simulink model "modelo_f_EXPORT_TO_CODESYS"  (R2024b)
settings: Solver=FixedStepAuto  StartTime=0.0  StopTime=inf  FixedStep=0.001  RelTol=1e-3  EnableMultiTasking=on
InitFcn:
  | clc
  | clear
  | close all
  | clear all
  | clear mex
  | parametros
  | gain_CL
  | calculo_observador_carro
  | calculo_observador_izaje
values from neighbouring files (symbols this model uses):
  b_cx = 1e6    (= 1000000)    [parametros.m]
  b_cy = 1e7    (= 10000000)    [parametros.m]
  b_hb = 1e8    (= 100000000)    [parametros.m]
  b_hd = 8    [parametros.m]
  b_hm = 18    [parametros.m]
  b_t = 90    [parametros.m]
  b_tb = 5e6    (= 5000000)    [parametros.m]
  b_td = 1.8    [parametros.m]
  b_tm = 6    [parametros.m]
  b_tw = 3e3    (= 3000)    [parametros.m]
  b_wu = 150    [parametros.m]
  container_pillars = container_pillars(randperm(19))    [parametros.m]
  dx_grid_lidar = 0.01    [parametros.m]
  escenario = 1    [parametros.m]
  g = 9.80665    [parametros.m]
  H_c = 2.59    [parametros.m]
  H_truck = 1    [parametros.m]
  i_h = 22    [parametros.m]
  i_t = 30    [parametros.m]
  J_hd_hEb = 3800    [parametros.m]
  J_hm_hb = 30    [parametros.m]
  J_td = 1200    [parametros.m]
  J_tm_tb = 7    [parametros.m]
  K_cy = 1.8e9    (= 1800000000)    [parametros.m]
  K_tw = 4.8e5    (= 480000)    [parametros.m]
  k_wu = 2.36e8    (= 236000000)    [parametros.m]
  l_h0 = (Y_t0-y_l0)    (= 38)    [parametros.m]
  l_h_max = Y_t0-y_h_min    (= 65)    [parametros.m]
  l_h_maxE = l_h_max+0.5    (= 65.5)    [parametros.m]
  l_h_min = Y_t0-y_h_max    (= 5)    [parametros.m]
  l_h_minE = l_h_min-0.5    (= 4.5)    [parametros.m]
  M_cmax = 50000    [parametros.m]
  M_cmin = 2000    [parametros.m]
  M_s = 15000    [parametros.m]
  M_t = 30000    [parametros.m]
  r_hd = 0.75    [parametros.m]
  r_td = 0.50    (= 0.5)    [parametros.m]
  T_hbMax = 5e4    (= 50000)    [parametros.m]
  T_hEbMax = 1.1e6    (= 1100000)    [parametros.m]
  T_hmMax = 2e4    (= 20000)    [parametros.m]
  T_s = 0.001    [parametros.m]
  T_s0 = 0.001    [parametros.m]
  T_s1 = 0.020    (= 0.02)    [parametros.m]
  T_s2 = 0.020    (= 0.02)    [parametros.m]
  T_tbMax = 5e3    (= 5000)    [parametros.m]
  T_tmMax = 4e3    (= 4000)    [parametros.m]
  tau_tm = 1e-3    (= 0.001)    [parametros.m]
  theta_hm0 = -l_h0*i_h*2/r_hd    (= -2229.33333333)    [parametros.m]
  theta_tm0 = (x_t0)*i_t/r_td    (= -900)    [parametros.m]
  trucks0 = [0, 0, 0, 0, 0]    [parametros.m]
  v_h_max_load = 1.5    [parametros.m]
  v_h_max_noload = 3    [parametros.m]
  v_lx0 = 0    [parametros.m]
  v_ly0 = 0    [parametros.m]
  v_t0 = 0    [parametros.m]
  v_t_max = 4    [parametros.m]
  W_c = ctrb(A, B_c(:,1))    [CyO_carro.m]    (also in CyO_izaje.m; parametros.m = 2.44)
  w_hm0 = 0    [parametros.m]
  w_hm_min_BRK = 0.005    [parametros.m]
  w_hm_rated = v_h_max_load*2*i_h/r_hd    (= 88)    [parametros.m]
  w_tm0 = (v_t0)*i_t/r_td    (= 0)    [parametros.m]
  w_tm_min_BRK = 0.005    [parametros.m]
  x_c0_left = -35    [parametros.m]
  x_c0_right = 55    [parametros.m]
  x_containers_left_lim = 1.5    [parametros.m]
  x_containers_right_lim = 48.5    [parametros.m]
  x_l0 = x_t0    (= -15)    [parametros.m]
  x_lidar_offset = 3.0    (= 3)    [parametros.m]
  x_t0 = -15    [parametros.m]
  x_t_max = 50    [parametros.m]
  x_t_maxE = x_t_max+0.5    (= 50.5)    [parametros.m]
  x_t_min = -30    [parametros.m]
  x_t_minE = x_t_min-0.5    (= -30.5)    [parametros.m]
  y_h_min = -20    [parametros.m]
  y_l0 = 7    [parametros.m]
  Y_sb = 5.0    (= 5)    [parametros.m]
  Y_t0 = 45    [parametros.m]
undefined symbols (not defined in the file or in its folder): parametros
libraries: dspnetwork x2, dspsigops x1, simulink x1
(part 4 of 4)

== stateflow chart modelo_f_EXPORT_TO_CODESYS/TO_CODESYS/Chart ==
  settings: executeAtInitialization=1
  state Nivel_1
    state Heartbeat_Generator [parallel]
      settings: executionOrder=1
      state Heartbeat_High
        entry:
        heartbeat = true;
      state Heartbeat_Low
        entry:
        heartbeat = false;
      (default) -> Heartbeat_High
      Heartbeat_Low -> Heartbeat_High : after(200, msec)
      Heartbeat_High -> Heartbeat_Low : after(200, msec)
    state SS_OFF [parallel]
      entry:
      BRK_h = false;
      BRK_t = false;
      TLK = false;
      v_t_ref = 0.0;
      dl_h_ref = 0.0;
      sway_ctr_enable = false;
      FC_t_min_alarm = false;
      FC_t_max_alarm = false;
      FC_h_min_alarm = false;
      FC_h_max_alarm = false;
      operation_mode = true;
      sway_ctr_gain = 1;
      container_pillars =zeros(1,19);
      m_est_vec = zeros(1, 500);
      m_est = 15000;
      trolley_moving = true;
      trolley_stopped = false;
      trolley_stopped_complete = false;
      hoist_moving = true;
      hoist_stopped = false;
      x_t_obj = x_t_est;
      x_t_ref = x_t_obj;
      l_h_obj = l_h_sensor;
      l_h_ref = l_h_obj;
      state_SISTEMA_ON = false;
      exit:
      state_SISTEMA_ON = true;
      x_t_pr = 0;
      l_h_pr = 0;
      v_t_ref_a = 0;
      dl_h_ref_a=0;
      settings: executionOrder=2
    state SS_ON [parallel]
      settings: executionOrder=3
      state BRK_Logic [parallel]
        settings: executionOrder=1
        state BRK_t_Logic [parallel]
          settings: executionOrder=1
          state BRK_t_Closed
            entry:
            BRK_t = false;
          state BRK_t_Opened
            entry:
            BRK_t = true;
          (default) -> BRK_t_Closed
          BRK_t_Opened -> BRK_t_Closed : [(abs(w_tm_estimada) > w_tm_min_BRK) &&  (FC_carro_min || FC_carro_max)]
          BRK_t_Closed -> BRK_t_Opened : [ ~(FC_carro_max && FC_carro_min) && x_t_est < (x_t_max-1.5) && x_t_est > (x_t_min+1.5)]
        state BRK_h_Logic [parallel]
          settings: executionOrder=2
          state BRK_h_Closed
            entry:
            BRK_h = false;
          state BRK_h_Opened
            entry:
            BRK_h = true;
          (default) -> BRK_h_Closed
          BRK_h_Opened -> BRK_h_Closed : [(abs(w_hm_estimada) > w_hm_min_BRK) && (FC_izaje_min || FC_izaje_max)]
          BRK_h_Closed -> BRK_h_Opened : [~(FC_izaje_max && FC_izaje_min) && l_h_sensor > (l_h_min + 1.5) && l_h_sensor < (l_h_max - 1.5)]
      state TLK_Logic [parallel]
        settings: executionOrder=2
        state Init
        state TLK_Opened
          entry:
          TLK = false;
        state TLK_Closed
          entry:
          TLK = true;
        (default) -> Nivel_1.SS_ON.TLK_Logic.Init
        Nivel_1.SS_ON.TLK_Logic.Init -> TLK_Closed [order 1] : [TLK]
        Nivel_1.SS_ON.TLK_Logic.Init -> TLK_Opened [order 2] : [~TLK]
        TLK_Opened -> TLK_Closed : [cmd_TLK && abs(F_hw_sensor) <= 0]
        TLK_Closed -> TLK_Opened : [~cmd_TLK && abs(F_hw_sensor) <= 0]
      state Sway_Control_Mode [parallel]
        settings: executionOrder=3
        state Sway_Control_ON
          entry:
          sway_ctr_enable = true;
        state Sway_Control_OFF
          entry:
          sway_ctr_enable = false;
        (default) -> Sway_Control_ON
        Sway_Control_ON -> Sway_Control_OFF : [~cmd_sway_ctr || l_h_sensor < 10]
        Sway_Control_OFF -> Sway_Control_ON : [cmd_sway_ctr && l_h_sensor > 11]
      state Lidar_Map [parallel]
        entry:
        land_end_element = floor((0 - x_c0_left)/dx_grid_lidar) + 1;
        land_end_element = max(1, min(lidar_grid_size, land_end_element));
        for idx = 1:9001
        if idx >= land_end_element
        lidar_map(idx) = y_h_min;
        end
        end
        cc = 0;
        during:
        x_lidar = x_t_est + x_lidar_offset;
        grid_element = max(1, min(lidar_grid_size, floor((x_lidar-x_c0_left)/dx_grid_lidar) + 1));
        lidar_map(grid_element) = y_c0_lidar;
        window_idx = round((v_t_max * T_s2) / dx_grid_lidar);
        n_pilares = 19;
        espaciado = (x_containers_right_lim - x_containers_left_lim) / (n_pilares - 1);
        l_h_safe = 45 - max(lidar_map) - 1.5 * H_c;
        for i = 1:n_pilares
        x_lidar_pillar = x_containers_left_lim + (i-1)*espaciado;
        grid_element_pillar = max(1, min(lidar_grid_size, floor((x_lidar_pillar - x_c0_left)/dx_grid_lidar) + 1));
        window_start = max(1, grid_element_pillar - window_idx);
        window_end   = min(lidar_grid_size, grid_element_pillar + window_idx);
        % --- REEMPLAZO PARA EVITAR ARREGLO DINAMICO ---
        pillar_height = lidar_map(window_start);
        for k = (window_start + 1):window_end
        if lidar_map(k) > pillar_height
        pillar_height = lidar_map(k);
        end
        end
        % ----------------------------------------------
        containers_height = pillar_height - y_h_min;
        container_pillars(i) = max(0, ceil(containers_height / H_c - 1e-6));
        end
        settings: executionOrder=5
      state Limit_Switch [parallel]
        during:
        settings: executionOrder=4
        state Trolley_Min_Logic [parallel]
          settings: executionOrder=1
          state FC_t_Min_High
            entry:
            FC_t_min_alarm = true;
          state FC_t_Min_Low
            entry:
            FC_t_min_alarm = false;
          (default) -> FC_t_Min_Low
          FC_t_Min_Low -> FC_t_Min_High : [FC_carro_min]
          FC_t_Min_High -> FC_t_Min_Low : [~FC_carro_min]
        state Trolley_Max_Logic [parallel]
          settings: executionOrder=2
          state FC_t_Max_High
            entry:
            FC_t_max_alarm = true;
          state FC_t_Max_Low
            entry:
            FC_t_max_alarm = false;
          (default) -> FC_t_Max_Low
          FC_t_Max_Low -> FC_t_Max_High : [FC_carro_max]
          FC_t_Max_High -> FC_t_Max_Low : [~FC_carro_max]
        state Hoist_Min_Logic [parallel]
          settings: executionOrder=3
          state FC_h_Min_High
            entry:
            FC_h_min_alarm = true;
          state FC_h_Min_Low
            entry:
            FC_h_min_alarm = false;
          (default) -> FC_h_Min_Low
          FC_h_Min_Low -> FC_h_Min_High : [FC_izaje_min]
          FC_h_Min_High -> FC_h_Min_Low : [~FC_izaje_min]
        state Hoist_Max_Logic [parallel]
          settings: executionOrder=4
          state FC_h_Max_Low
            entry:
            FC_h_max_alarm = false;
          state FC_h_Max_High
            entry:
            FC_h_max_alarm = true;
          (default) -> FC_h_Max_Low
          FC_h_Max_Low -> FC_h_Max_High : [FC_izaje_max]
          FC_h_Max_High -> FC_h_Max_Low : [~FC_izaje_max]
      state Trolley_Movement_Flags [parallel]
        settings: executionOrder=8
        state Trolley_Moving
          entry:
          trolley_moving = true;
          trolley_stopped = false;
          trolley_stopped_complete = false;
        state Trolley_Stopped
          entry:
          trolley_moving = false;
          trolley_stopped = true;
          trolley_stopped_complete = false;
        state Trolley_Stopped_Complete
          entry:
          trolley_moving = false;
          trolley_stopped = true;
          trolley_stopped_complete = true;
        (default) -> Trolley_Moving
        Trolley_Moving -> Trolley_Stopped : [abs(x_t_est-x_t_obj) <= 0.03 && abs(v_t_est) <= 0.05]
        Trolley_Stopped_Complete -> Trolley_Moving [order 2] : [abs(x_t_est-x_t_obj) > 0.15 || abs(v_t_est) > 0.15]
        Trolley_Stopped -> Trolley_Moving [order 1] : [abs(x_t_est-x_t_obj) > 0.1 || abs(v_t_est) > 0.1]
        Trolley_Stopped -> Trolley_Stopped_Complete [order 2] : [abs(w_l_sensor) <= 0.005 && abs(theta_l_sensor) <= 0.005]
        Trolley_Stopped_Complete -> Trolley_Stopped [order 1] : [abs(w_l_sensor) > 0.01 || abs(theta_l_sensor) > 0.01]
      state Hoist_Movement_Flags [parallel]
        settings: executionOrder=9
        state Hoist_Stopped
          entry:
          hoist_moving = false;
          hoist_stopped = true;
        state Hoist_Moving
          entry:
          hoist_moving = true;
          hoist_stopped = false;
        (default) -> Hoist_Moving
        Hoist_Stopped -> Hoist_Moving : [abs(l_h_sensor-l_h_obj) > 0.1 || abs(dl_h_est) > 0.1]
        Hoist_Moving -> Hoist_Stopped : [abs(l_h_sensor-l_h_obj) <= 0.05 && abs(dl_h_est) <= 0.05]
      state Mode [parallel]
        settings: executionOrder=6
        state Automatic
          during:
        state Manual
          entry:
          v_t_ref_prev = v_t_ref;
          dl_h_ref_prev = dl_h_ref;
          x_t_ref = x_t_est;
          l_h_ref = l_h_sensor;
          during:
          %...v_t_ref_a = rate_limiter(JS_trolley_cmd*0.15, v_t_ref_prev, 0, T_s1, m_est);
          %...dl_h_ref_a = rate_limiter(JS_hoist_cmd*0.15, dl_h_ref_prev, 1, T_s1, m_est);
          if FC_t_min_alarm
          v_t_ref = max([0, v_t_ref_a]);
          elseif FC_t_max_alarm
          v_t_ref = min([0, v_t_ref_a]);
          else
          v_t_ref = v_t_ref_a;
          end
          if FC_h_min_alarm
          dl_h_ref = max([0, dl_h_ref_a]);
          elseif FC_h_max_alarm
          dl_h_ref = min([0, dl_h_ref_a]);
          else
          dl_h_ref = dl_h_ref_a;
          end
          x_t_ref = x_t_ref + T_s1 * (v_t_ref + v_t_ref_prev)/2;
          l_h_ref = l_h_ref + T_s1 * (dl_h_ref + dl_h_ref_prev)/2;
          v_t_ref_prev = v_t_ref;
          dl_h_ref_prev = dl_h_ref;
        (default) -> Automatic
        Manual -> Automatic : [operation_mode]
        Automatic -> Manual : [~operation_mode]
      state Trajectory_Planner [parallel]
        settings: executionOrder=7
        state Line_Scan_Rise
          entry:
          l_h_obj = l_h_safe;
          %...[l_h_ref, dl_h_ref, ~, l_h_pr] = generador_trayectoria_izaje(t, l_h_sensor, v_t_est, l_h_obj, m_est, 1);
          during:
          %...[l_h_ref, dl_h_ref, ~, l_h_pr] = generador_trayectoria_izaje(t, l_h_sensor, v_t_est, l_h_obj, m_est, 0);
        state Scenario_Selector
          entry:
          sway_ctr_gain = 1;
        state Waiting
          entry:
          v_t_ref  = 0;
          dl_h_ref = 0;
        state Line_Scan_Move
          entry:
          x_t_obj = 49.5;
          %...[x_t_ref, v_t_ref, ~, x_t_pr] = generador_trayectoria(t, x_t_est, x_t_obj, v_t_est, 1);
          during:
          %...[x_t_ref, v_t_ref, ~, x_t_pr] = generador_trayectoria(t, x_t_est, x_t_obj, v_t_est, 0);
          %...[l_h_ref, dl_h_ref, ~, l_h_pr] = generador_trayectoria_izaje(t, l_h_sensor, v_t_est, l_h_obj, m_est, 0);
        state Pickup_And_Place_Loop
          exit:
          loop_initialized = true;
          state Init
          state Scenario_Selector
          state Truck_Pickup_Raise
            entry:
            operation_mode = true;
            l_h_obj = l_h_safe;
            %...[l_h_ref, dl_h_ref, ~, l_h_pr] = generador_trayectoria_izaje(t, l_h_sensor, v_t_est, l_h_obj, m_est, 1);
            during:
            %...[l_h_ref, dl_h_ref, ~, l_h_pr] = generador_trayectoria_izaje(t, l_h_sensor, v_t_est, l_h_obj, m_est, 0);
            %...[x_t_ref, v_t_ref, ~, x_t_pr] = generador_trayectoria(t, x_t_est, x_t_obj, v_t_est, 0);
          state Truck_Placement_Manual
            entry:
            operation_mode = false;
            exit:
            m_est = 15000;
          state Truck_Pickup_Move
            entry:
            operation_mode = true;
            for i = 1:5
            if trucks_state(i) == 1
            if trucks_has_load(i) == 1
            x_t_obj = -25 + (i-1)*5;
            end
            end
            end
            x_t_obj
            %...[x_t_ref, v_t_ref, ~, x_t_pr] = generador_trayectoria(t, x_t_est, x_t_obj, v_t_est, 1);
            during:
            %...[x_t_ref, v_t_ref, ~, x_t_pr] = generador_trayectoria(t, x_t_est, x_t_obj, v_t_est, 0);
            %...[l_h_ref, dl_h_ref, ~, l_h_pr] = generador_trayectoria_izaje(t, l_h_sensor, v_t_est, l_h_obj, m_est, 0);
          state Truck_Placement_Descend
            entry:
            operation_mode = true;
            l_h_obj = 45 - truck_pickup_height - pickup_safety_margin
            %...[l_h_ref, dl_h_ref, ~, l_h_pr] = generador_trayectoria_izaje(t, l_h_sensor, v_t_est, l_h_obj, m_est, 1);
            during:
            %...[l_h_ref, dl_h_ref, ~, l_h_pr] = generador_trayectoria_izaje(t, l_h_sensor, v_t_est, l_h_obj, m_est, 0);
            %...[x_t_ref, v_t_ref, ~, x_t_pr] = generador_trayectoria(t, x_t_est, x_t_obj, v_t_est, 0);
          state Truck_Placement_Move
            entry:
            operation_mode = true;
            for i = 1:5
            if trucks_state(i) == 1
            if trucks_has_load(i) == 0
            x_t_obj = -25 + (i-1)*5;
            end
            end
            end
            x_t_obj
            %...[x_t_ref, v_t_ref, ~, x_t_pr] = generador_trayectoria(t, x_t_est, x_t_obj, v_t_est, 1);
            during:
            %...[x_t_ref, v_t_ref, ~, x_t_pr] = generador_trayectoria(t, x_t_est, x_t_obj, v_t_est, 0);
            %...[l_h_ref, dl_h_ref, ~, l_h_pr] = generador_trayectoria_izaje(t, l_h_sensor, v_t_est, l_h_obj, m_est, 0);
          state Truck_Pickup_Descend
            entry:
            operation_mode = true;
            l_h_obj = 45 - truck_pickup_height - pickup_safety_margin
            %...[l_h_ref, dl_h_ref, ~, l_h_pr] = generador_trayectoria_izaje(t, l_h_sensor, v_t_est, l_h_obj, m_est, 1);
            during:
            %...[l_h_ref, dl_h_ref, ~, l_h_pr] = generador_trayectoria_izaje(t, l_h_sensor, v_t_est, l_h_obj, m_est, 0);
            %...[x_t_ref, v_t_ref, ~, x_t_pr] = generador_trayectoria(t, x_t_est, x_t_obj, v_t_est, 0);
          state Truck_Placement_Raise
            entry:
            operation_mode = true;
            l_h_obj = l_h_safe;
            %...[l_h_ref, dl_h_ref, ~, l_h_pr] = generador_trayectoria_izaje(t, l_h_sensor, v_t_est, l_h_obj, m_est, 1);
            during:
            %...[l_h_ref, dl_h_ref, ~, l_h_pr] = generador_trayectoria_izaje(t, l_h_sensor, v_t_est, l_h_obj, m_est, 0);
            %...[x_t_ref, v_t_ref, ~, x_t_pr] = generador_trayectoria(t, x_t_est, x_t_obj, v_t_est, 0);
          state Truck_Pickup_Manual
            entry:
            operation_mode = false;
            m_est_vec_pos = 1;
            m_est_vec(:) = 0;
            during:
            if F_hw_sensor > 8000*g && m_est_vec_pos <= length(m_est_vec(1,:))
            m_est_vec(1, m_est_vec_pos) = 2*F_hw_sensor/g;
            m_est_vec_pos = m_est_vec_pos + 1;
            end
            exit:
            %... m_est = estimar_masa(m_est_vec);
          state Ship_Pickup_Manual
            entry:
            operation_mode = false;
            m_est_vec_pos = 1;
            m_est_vec(:) = 0;
            during:
            if F_hw_sensor > 8000*g && m_est_vec_pos <= length(m_est_vec(1,:))
            m_est_vec(1, m_est_vec_pos) = 2*F_hw_sensor/g;
            m_est_vec_pos = m_est_vec_pos + 1;
            end
            exit:
            %...m_est = estimar_masa(m_est_vec);
          state Ship_Placement_Raise
            entry:
            operation_mode = true;
            l_h_obj = l_h_safe;
            %...[l_h_ref, dl_h_ref, ~, l_h_pr] = generador_trayectoria_izaje(t, l_h_sensor, v_t_est, l_h_obj, m_est, 1);
            during:
            %...[l_h_ref, dl_h_ref, ~, l_h_pr] = generador_trayectoria_izaje(t, l_h_sensor, v_t_est, l_h_obj, m_est, 0);
            %...[x_t_ref, v_t_ref, ~, x_t_pr] = generador_trayectoria(t, x_t_est, x_t_obj, v_t_est, 0);
          state Ship_Pickup_Descend
            entry:
            operation_mode = true;
            %...l_h_obj = xpos2ypos(lidar_map, x_t_obj) - placement_safety_margin
            %...[l_h_ref, dl_h_ref, ~, l_h_pr] = generador_trayectoria_izaje(t, l_h_sensor, v_t_est, l_h_obj, m_est, 1);
            during:
            %...[l_h_ref, dl_h_ref, ~, l_h_pr] = generador_trayectoria_izaje(t, l_h_sensor, v_t_est, l_h_obj, m_est, 0);
            %...[x_t_ref, v_t_ref,  ~, x_t_pr] = generador_trayectoria(t, x_t_est, x_t_obj, v_t_est, 0);
          state Ship_Placement_Move
            entry:
            operation_mode = true;
            min_containers = 999;
            idx_obj = 1;
            for i = 1:19
            if container_pillars(i) < min_containers
            min_containers = container_pillars(i);
            idx_obj = i;
            end
            end
            espaciado = (x_containers_right_lim - x_containers_left_lim) / (19 - 1);
            x_t_obj = x_containers_left_lim + (idx_obj - 1) * espaciado;
            x_t_obj
            %...[x_t_ref, v_t_ref, ~, x_t_pr] = generador_trayectoria(t, x_t_est, x_t_obj, v_t_est,1 );
            during:
            %...[x_t_ref, v_t_ref,  ~, x_t_pr] = generador_trayectoria(t, x_t_est, x_t_obj, v_t_est, 0);
            %...[l_h_ref, dl_h_ref, ~, l_h_pr] = generador_trayectoria_izaje(t, l_h_sensor, v_t_est, l_h_obj, m_est, 0);
          state Ship_Pickup_Move
            entry:
            operation_mode = true;
            max_containers = 0;
            idx_obj = 1;
            for i = 1:19
            if container_pillars(i) > max_containers
            max_containers = container_pillars(i);
            idx_obj = i;
            end
            end
            espaciado = (x_containers_right_lim - x_containers_left_lim) / (19 - 1);
            x_t_obj = x_containers_left_lim + (idx_obj - 1) * espaciado;
            x_t_obj
            %...[x_t_ref, v_t_ref, ~, x_t_pr] = generador_trayectoria(t, x_t_est, x_t_obj, v_t_est,1 );
            during:
            %...[x_t_ref, v_t_ref,  ~, x_t_pr] = generador_trayectoria(t, x_t_est, x_t_obj, v_t_est, 0);
            %...[l_h_ref, dl_h_ref, ~, l_h_pr] = generador_trayectoria_izaje(t, l_h_sensor, v_t_est, l_h_obj, m_est, 0);
          state Ship_Palcement_Descend
            entry:
            operation_mode = true;
            %...l_h_obj = xpos2ypos(lidar_map, x_t_obj) - placement_safety_margin
            %...[l_h_ref, dl_h_ref, ~, l_h_pr] = generador_trayectoria_izaje(t, l_h_sensor, v_t_est, l_h_obj, m_est, 1);
            during:
            %...[l_h_ref, dl_h_ref, ~, l_h_pr] = generador_trayectoria_izaje(t, l_h_sensor, v_t_est, l_h_obj, m_est, 0);
            %...[x_t_ref, v_t_ref,  ~, x_t_pr] = generador_trayectoria(t, x_t_est, x_t_obj, v_t_est, 0);
          state Ship_Pickup_Raise
            entry:
            operation_mode = true;
            l_h_obj = l_h_safe;
            %...[l_h_ref, dl_h_ref, ~, l_h_pr] = generador_trayectoria_izaje(t, l_h_sensor, v_t_est, l_h_obj, m_est, 1);
            during:
            %...[l_h_ref, dl_h_ref, ~, l_h_pr] = generador_trayectoria_izaje(t, l_h_sensor, v_t_est, l_h_obj, m_est, 0);
            %...[x_t_ref, v_t_ref, ~, x_t_pr] = generador_trayectoria(t, x_t_est, x_t_obj, v_t_est, 0);
          state Ship_Placement_Manual
            entry:
            operation_mode = false;
            exit:
            m_est = 15000;
          (default) -> Nivel_1.SS_ON.Trajectory_Planner.Pickup_And_Place_Loop.Init
          Nivel_1.SS_ON.Trajectory_Planner.Pickup_And_Place_Loop.Init -> (history) [order 2] : [loop_initialized]
          Nivel_1.SS_ON.Trajectory_Planner.Pickup_And_Place_Loop.Init -> Nivel_1.SS_ON.Trajectory_Planner.Pickup_And_Place_Loop.Scenario_Selector [order 1] : [~loop_initialized]
          Nivel_1.SS_ON.Trajectory_Planner.Pickup_And_Place_Loop.Scenario_Selector -> Ship_Pickup_Raise [order 2] : [escenario == 2]
          Nivel_1.SS_ON.Trajectory_Planner.Pickup_And_Place_Loop.Scenario_Selector -> Truck_Pickup_Raise [order 1] : [escenario == 1 || escenario == 3]
          Truck_Placement_Manual -> Truck_Pickup_Move [order 2] : [(l_h_sensor <=  l_h_obj-1 && ~TLK) && escenario == 3]
          Truck_Placement_Manual -> Ship_Pickup_Raise [order 1] : [(l_h_sensor <=  l_h_obj-1 && ~TLK) && escenario == 2]
          Truck_Placement_Descend -> Truck_Placement_Manual : [hoist_stopped && trolley_stopped_complete]
          Truck_Pickup_Raise -> Truck_Pickup_Move : [hoist_stopped || l_h_pr > 0.8]
          Ship_Placement_Manual -> Truck_Pickup_Raise [order 1] : [(l_h_sensor <=  l_h_obj-1 && ~TLK) && escenario == 1]
          Truck_Placement_Move -> Truck_Placement_Descend : [trolley_stopped]
          Truck_Pickup_Move -> Truck_Pickup_Descend : [trolley_stopped_complete || x_t_pr > 0.95]
          Truck_Placement_Raise -> Truck_Placement_Move : [hoist_stopped || l_h_pr > 0.8]
          Truck_Pickup_Descend -> Truck_Pickup_Manual : [hoist_stopped && trolley_stopped_complete]
          Ship_Pickup_Manual -> Truck_Placement_Raise : [l_h_sensor <=  l_h_obj-1 && TLK]
          Truck_Pickup_Manual -> Ship_Placement_Raise : [l_h_sensor <= l_h_obj-1 && TLK]
          Ship_Pickup_Descend -> Ship_Pickup_Manual : [hoist_stopped]
          Ship_Placement_Raise -> Ship_Placement_Move : [hoist_stopped || l_h_pr > 0.8]
          Ship_Pickup_Move -> Ship_Pickup_Descend : [trolley_stopped_complete]
          Ship_Placement_Move -> Ship_Palcement_Descend : [trolley_stopped_complete]
          Ship_Pickup_Raise -> Ship_Pickup_Move : [hoist_stopped || l_h_pr > 0.8]
          Ship_Palcement_Descend -> Ship_Placement_Manual : [hoist_stopped]
          Ship_Placement_Manual -> Ship_Pickup_Raise [order 2] : [([l_h_sensor <=  l_h_obj-1 && ~TLK]) && escenario == 3]
        state Line_Scan_Return
          entry:
          x_t_obj = -29.5;
          %...[x_t_ref, v_t_ref, ~, x_t_pr] = generador_trayectoria(t, x_t_est, x_t_obj, v_t_est, 1);
          during:
          %...[x_t_ref, v_t_ref, ~, x_t_pr] = generador_trayectoria(t, x_t_est, x_t_obj, v_t_est, 0);
          %...[l_h_ref, dl_h_ref, ~, l_h_pr] = generador_trayectoria_izaje(t, l_h_sensor, v_t_est, l_h_obj, m_est, 0);
        (default) -> Line_Scan_Rise
        Nivel_1.SS_ON.Trajectory_Planner.Scenario_Selector -> Waiting [order 1] : [escenario == 0]
        Line_Scan_Return -> Nivel_1.SS_ON.Trajectory_Planner.Scenario_Selector : [trolley_stopped && hoist_stopped]
        Waiting -> Nivel_1.SS_ON.Trajectory_Planner.Scenario_Selector : [escenario ~= 0]
        Line_Scan_Rise -> Line_Scan_Move : [hoist_stopped || l_h_pr > 0.8]
        Pickup_And_Place_Loop -> Nivel_1.SS_ON.Trajectory_Planner.Scenario_Selector : [FC_t_min_alarm || FC_t_max_alarm || FC_h_min_alarm || FC_h_max_alarm]
        Nivel_1.SS_ON.Trajectory_Planner.Scenario_Selector -> Pickup_And_Place_Loop [order 2] : [escenario ~= 0]
        Line_Scan_Move -> Line_Scan_Return : [trolley_stopped]
    (default) -> SS_OFF
    SS_OFF -> SS_ON : [P_APN ]
    SS_ON -> SS_OFF : [~P_APN || emgy || P_E]
  (default) -> Nivel_1
  data: emgy input boolean size=1; v_t_ref output double size=1 =0; BRK_h output boolean size=1; theta_l_sensor input double size=1; w_l_sensor input double size=1; w_tm_estimada input double size=1; JS_trolley_cmd input double size=1; JS_hoist_cmd input double size=1; w_hm_estimada input double size=1; y_c0_lidar input double size=1; P_APN input boolean size=1; P_E input boolean size=1; dl_h_est input double size=1; cmd_sway_ctr input boolean size=1; trucks_state input double size=1,5; trucks_has_load input double size=1,5; l_h_sensor input double size=1; FC_izaje_min input boolean size=1; FC_izaje_max input boolean size=1; FC_carro_max input boolean size=1; FC_carro_min input boolean size=1; cmd_TLK input boolean size=1; F_hw_sensor input double size=1; w_hm_min_BRK parameter double size=1; w_tm_min_BRK parameter double size=1; sway_ctr_enable output boolean size=1; dl_h_ref output double size=1; heartbeat output boolean size=1; l_h_max parameter double size=1; x_t_max parameter double size=1; x_t_min parameter double size=1; x_t_est input double size=1; x_lidar_offset parameter double size=1; dx_grid_lidar parameter double size=1; x_lidar local double size=1; grid_element local double size=1; lidar_map local double size=9001; TLK output boolean size=1 =false; v_t_est input double size=1; v_t_max constant double size=1 =v_t_max; v_t_ref_prev local double size=1 =0; T_s2 constant double size=1 =T_s2; x_t_obj local double size=1; sway_ctr_gain output double size=1 =1; escenario constant double size=1 =escenario; i local double size=1; x_c0_left constant double size=1 =x_c0_left; container_pillars local double size=1,19; lidar_grid_size constant double size=1 =lidar_grid_size; x_lidar_pillar local double size=1; grid_element_pillar local double size=1; y_h_min constant double size=1 =y_h_min; H_c constant double size=1 =H_c; containers_height local double size=1; land_end_element local double size=1; window_idx local double size=1; window_end local double size=1; window_start local double size=1; pillar_height local double size=1; idx_obj local double size=1; min_containers local double size=1; l_h_obj local double size=1; x_t_ref output double size=1; truck_pickup_height constant double size=1 =truck_pickup_height; trolley_moving local boolean size=1; trolley_stopped_complete local boolean size=1; trolley_stopped local boolean size=1; l_h_ref output double size=1 =l_h0; pickup_safety_margin constant double size=1 =pickup_safety_margin; hoist_moving local boolean size=1; hoist_stopped local boolean size=1; x_containers_left_lim constant double size=1 =x_containers_left_lim; x_containers_right_lim constant double size=1 =x_containers_right_lim; n_pilares local double size=1; espaciado local double size=1; cc local double size=1; l_h_safe local double size=1 =13; operation_mode output boolean size=1 =1; dl_h_ref_prev local double size=1; T_s1 local double size=1 =T_s1; l_h_pr local double size=1; x_t_pr local double size=1; BRK_t output boolean size=1; m_est output double size=1 =15000; m_est_vec local double size=1,500; m_est_vec_pos local double size=1; g constant double size=1 =g; l_h_min local double size=1 =l_h_min; max_containers local double size=1 =0; dl_h_ref_a local double size=1; v_t_ref_a local double size=1; loop_initialized local boolean size=1 =false; state_SISTEMA_ON output boolean size=1 =false; FC_h_max_alarm output boolean size=1 =false; FC_h_min_alarm output boolean size=1 =false; FC_t_max_alarm output boolean size=1 =false; FC_t_min_alarm output boolean size=1 =false; idx local double size=1 =1; k local double size=1
